simulink model "chaotic_freq_spring"  (Simulink 6.6)
settings: Solver=ode4  StartTime=h  StopTime=80  FixedStep=h  RelTol=1e-3
undefined symbols (not defined in the file): a, b, c, g, k, tau
settings Model: Creator=stepp  LastModifiedBy=stepp  ExtModeAutoUpdateStatusClock=off
settings DataIOCC: LimitDataPoints=off  SaveState=on  SignalLogging=off  StateSaveName=x  TimeSaveName=t  OutputSaveName=y

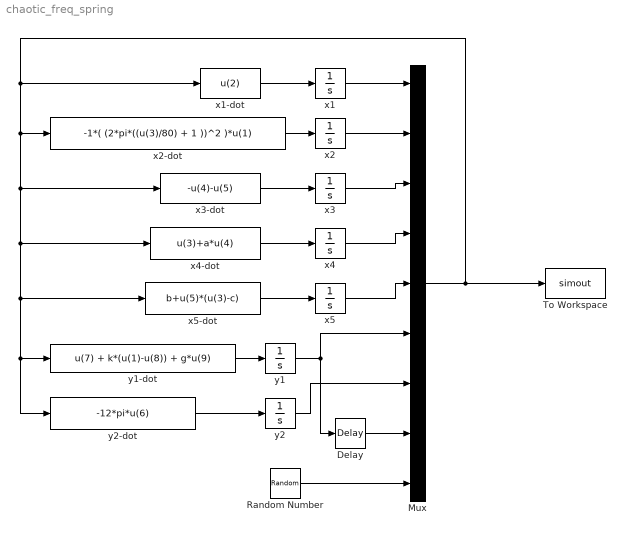
== system chaotic_freq_spring ==
  Delay : TransportDelay  DelayTime=tau
  Mux : Mux  Inputs=9
  Random Number : RandomNumber  SampleTime=0
  To Workspace : ToWorkspace  VariableName=simout  SampleTime=-1  SaveFormat=Array
  x1 : Integrator  InitialCondition=1
  x1-dot : Fcn  Expr=u(2)
  x2 : Integrator
  x2-dot : Fcn  Expr=-1*( (2*pi*((u(3)/80) + 1 ))^2 )*u(1)
  x3 : Integrator  InitialCondition=18.68
  x3-dot : Fcn  Expr=-u(4)-u(5)
  x4 : Integrator  InitialCondition=3.432
  x4-dot : Fcn  Expr=u(3)+a*u(4)
  x5 : Integrator  InitialCondition=20.9
  x5-dot : Fcn  Expr=b+u(5)*(u(3)-c)
  y1 : Integrator  InitialCondition=1
  y1-dot : Fcn  Expr=u(7) + k*(u(1)-u(8)) + g*u(9)
  y2 : Integrator
  y2-dot : Fcn  Expr=-12*pi*u(6)
  wires:
  x1-dot/1 -> x1/1
  x2-dot/1 -> x2/1
  x3-dot/1 -> x3/1
  x4-dot/1 -> x4/1
  x5-dot/1 -> x5/1
  x1/1 -> Mux/1
  x2/1 -> Mux/2
  x3/1 -> Mux/3
  x4/1 -> Mux/4
  x5/1 -> Mux/5
  Mux/1 -> x1-dot/1, x2-dot/1, x3-dot/1, x4-dot/1, x5-dot/1, y1-dot/1, y2-dot/1, To Workspace/1
  y2-dot/1 -> y2/1
  y1-dot/1 -> y1/1
  y1/1 -> Delay/1, Mux/6
  Delay/1 -> Mux/8
  y2/1 -> Mux/7
  Random Number/1 -> Mux/9
